simulink model "brasonduleur1"  (Simulink 7.9)
settings: Solver=ode1  StartTime=0.0  StopTime=1  RelTol=1e-3
libraries: powerlib x19, powerlib_extras x7, simulink_extras x1
settings Model: Creator=LiberT  LastModifiedBy=LiberT

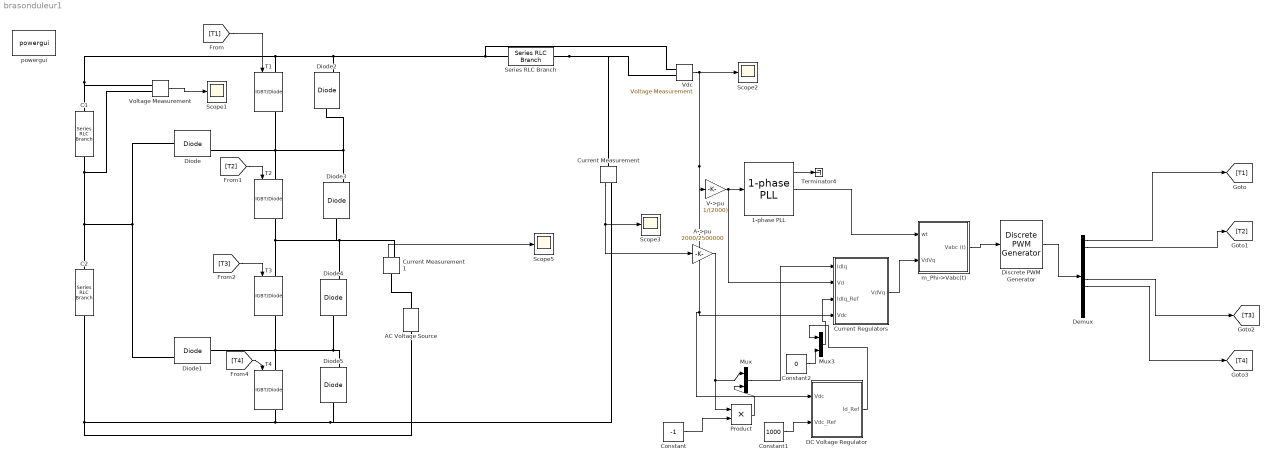
== system brasonduleur1 ==
  1-phase PLL : powerlib_extras/Control  Blocks/1-phase PLL  Par_Init=[0 60]  ParK=[ 180 3200 1 ]  AGC=off
  A->pu : Gain  Gain=2000/2500000  SaturateOnIntegerOverflow=on  OutDataTypeStr=Inherit: Same as input  ParamDataTypeStr=Inherit: Same as input
  AC Voltage Source : powerlib/Electrical Sources/AC Voltage Source  Amplitude=2e3  Phase=0  Frequency=60  SampleTime=0  Measurements=None
  C1 : powerlib/Elements/Series RLC Branch  LConnTagsString=__new0  RConnTagsString=__new0  BranchType=C  Resistance=1  Inductance=1e-3  SetiL0=off  InitialCurrent=0  Capacitance=150e-5  Setx0=off  InitialVoltage=0  Measurements=None
  C2 : powerlib/Elements/Series RLC Branch  LConnTagsString=__new0  RConnTagsString=__new0  BranchType=C  Resistance=1  Inductance=1e-3  SetiL0=off  InitialCurrent=0  Capacitance=150e-5  Setx0=off  InitialVoltage=0  Measurements=None
  Constant : Constant  Value=-1
  Constant1 : Constant  Value=1000
  Constant2 : Constant  Value=0
  Current Regulators : Subsystem  mask(Current Regulators){Kp=0.3, Ki=20, Kd=0, TcD=0.2e-3, Par_Limits=[12 -12], Init=0, Ts=5e-6}
      mask prompts: Kp "Proportional gain (Kp):"; Ki "Integral gain (Ki):"; Kd "Derivative gain (Kd):"; TcD "Time constant for derivative (s):"; Par_Limits "Output limits: [ Upper   Lower ]"; Init "Output initial value:"; Ts "Sample time:"
      mask help:
      | Sign convention:
      | Id positive(+) flowing into converter ==> Converter absorbing real power = P positive(+)
      | Iq negative(-) flowing into converter (inductive current) ==> Converter absorbing reactive power = Q positive(+)
  Current Measurement : powerlib/Measurements/Current Measurement  PhasorSimulation=off  OutputType=Complex  PSBequivalent=0
  Current Measurement1 : powerlib/Measurements/Current Measurement  PhasorSimulation=off  OutputType=Complex  PSBequivalent=0
  DC Voltage Regulator : Subsystem  mask(DC Voltage regulator){Kp=0.015, Ki=1.6, Ts=5e-6}
      mask prompts: Kp "Proportional gain (Kp):"; Ki "Integral gain(Ki)"; Ts "Sample time:"
  Demux : Demux  Outputs=12
  Diode{,1..5} (6 alike) : powerlib/Power Electronics/Diode  Ron=0.001  Lon=0  Vf=0.8  IC=0  UseSnubber=off  Rs=500  Cs=250e-9  Measurements=on
  Discrete PWM Generator : powerlib_extras/Discrete  Control Blocks/Discrete PWM Generator  GeneratorMode="Double 3-arm  bridges (12 pulses)"  Fc=333  Ts=5e-6  Internal=off  mIndex=0.4  Freq=333  Phase=0
  Mux : Mux  Inputs=2
  Mux3 : Mux  Inputs=2
  Product : Product  RndMeth=Zero
  Scope{1..3,5} (4 alike) : Scope
      Scope1 settings: YMin=1037.25  YMax=1041.5
      Scope2 settings: YMin=-1750  YMax=2500
      Scope3 settings: YMin=0.0965  YMax=0.1015  SaveName=ScopeData2
      Scope5 settings: YMin=-27500  YMax=2500  SaveName=ScopeData4
  Series RLC Branch : powerlib/Elements/Series RLC Branch  LConnTagsString=__new0  RConnTagsString=__new0  BranchType=RL  Resistance=1.25  Inductance=1  SetiL0=off  InitialCurrent=0  Capacitance=0  Setx0=off  InitialVoltage=0  Measurements=None
  T{1..4} (4 alike) : powerlib/Power Electronics/IGBT//Diode  Ron=0.2e-3  Rs=50  Cs=1e-6  Measurements=on
  Terminator4 : Terminator
  V->pu : Gain  Gain=1/(2000)  SaturateOnIntegerOverflow=on  OutDataTypeStr=Inherit: Same as input  ParamDataTypeStr=Inherit: Same as input
  Vdc : powerlib/Measurements/Voltage Measurement  PhasorSimulation=off  OutputType=Complex  PSBequivalent=0
  Voltage Measurement : powerlib/Measurements/Voltage Measurement  PhasorSimulation=off  OutputType=Complex  PSBequivalent=0
  m_Phi->Vabc(t) : Subsystem
  powergui : powerlib/powergui  Priority=1  SimulationMode=Discrete  SolverType=Tustin  SampleTime=50e-7  frequency=60  SPID=off  DisableSnubberDevices=off  DisableRonSwitches=off  DisableVfSwitches=off  SwTol=0  Interpol=off  DisplayEquations=off  FunctionMessages=off  frequencyindice=0  Pbase=100e6  ErrMax=1e-4  Iterations=50  UnitsV=kV  UnitsW=MW  echomessages=off  HookPort=off  EnableUseOfTLC=off  x0status=blocks  RestoreLinks=warning  ResistiveCurrentMeasurement=off  Ylog=off  Xlog=on  ShowGrid=off  save=off  variable=ZData  ZoomFFT=off  StartTime=0.0  cycles=1  DisplayStyle=1  FreqAxis=off  MaxFrequency=1000  frequencyindicesteady=1  display=off  methode=off
  wires:
  [T4] -> T4/1
  [T2] -> T2/1
  [T1] -> T1/1
  [T3] -> T3/1
  Voltage Measurement/1 -> Scope1/1
  Demux/2 -> [T2]
  Demux/8 -> [T4]
  Demux/7 -> [T3]
  Vdc/1 -> Scope2/1, V->pu/1, Current Regulators/4(Vdc), DC Voltage Regulator/1(Vdc)
  Current Measurement/1 -> Scope3/1, A->pu/1
  Demux/1 -> [T1]
  V->pu/1 -> 1-phase PLL/1, Current Regulators/2(Vd)
  1-phase PLL/1 -> Terminator4/1
  A->pu/1 -> Product/1, Mux/1
  Constant/1 -> Product/2
  Product/1 -> Mux/2
  Mux/1 -> Current Regulators/1(IdIq)
  Constant1/1 -> DC Voltage Regulator/2(Vdc_Ref)
  Constant2/1 -> Mux3/2
  DC Voltage Regulator/1(Id_Ref) -> Mux3/1
  Mux3/1 -> Current Regulators/3(IdIq_Ref)
  Current Regulators/1(VdVq) -> m_Phi->Vabc(t)/2(VdVq)
  1-phase PLL/2 -> m_Phi->Vabc(t)/1(wt)
  m_Phi->Vabc(t)/1(Vabc (t)) -> Discrete PWM Generator/1
  Current Measurement1/1 -> Scope5/1
  Discrete PWM Generator/1 -> Demux/1
  connections:
  Diode5/RConn1 -- T3/RConn1 -- T4/LConn1 -- Diode1/LConn1 -- Diode4/LConn1
  T1/RConn1 -- T2/LConn1 -- Diode/RConn1 -- Diode3/RConn1 -- Diode2/LConn1
  Series RLC Branch/LConn1 -- Vdc/LConn1 -- Diode2/RConn1 -- C1/LConn1 -- Voltage Measurement/LConn1 -- T1/LConn1
  C2/RConn1 -- T4/RConn1 -- Diode5/LConn1 -- Current Measurement/RConn1 -- AC Voltage Source/LConn1
  C1/RConn1 -- C2/LConn1 -- Diode1/RConn1 -- Diode/LConn1 -- Voltage Measurement/LConn2
  Series RLC Branch/RConn1 -- Current Measurement/LConn1 -- Vdc/LConn2
  T2/RConn1 -- T3/LConn1 -- Current Measurement1/RConn1 -- Diode4/RConn1 -- Diode3/LConn1
  AC Voltage Source/RConn1 -- Current Measurement1/LConn1

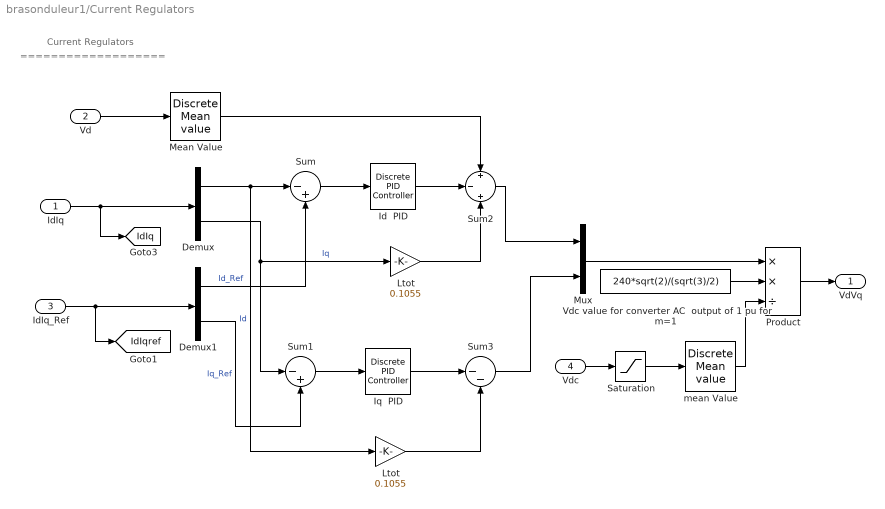
== system brasonduleur1/Current Regulators ==
  note: ===================
  note: Current Regulators
  IdIq : Inport  PortDimensions=2
  Vd : Inport  Port=2
  IdIq_Ref : Inport  Port=3  PortDimensions=2
  Vdc : Inport  Port=4
  " Ltot" : Gain  Gain=0.1055  SaturateOnIntegerOverflow=on  OutDataTypeStr=Inherit: Same as input  ParamDataTypeStr=Inherit: Same as input
  Demux : Demux  Outputs=2
  Demux1 : Demux  Outputs=2
  Id  PID : powerlib_extras/Discrete  Control Blocks/Discrete PID Controller  Kp=Kp  Ki=Ki  Kd=Kd  TcD=TcD  Par_Limits=Par_Limits  Init=Init  Ts=Ts
  Iq  PID : powerlib_extras/Discrete  Control Blocks/Discrete PID Controller  Kp=Kp  Ki=Ki  Kd=Kd  TcD=TcD  Par_Limits=Par_Limits  Init=Init  Ts=Ts
  "Ltot " : Gain  Gain=0.1055  SaturateOnIntegerOverflow=on  OutDataTypeStr=Inherit: Same as input  ParamDataTypeStr=Inherit: Same as input
  Mean Value : powerlib_extras/Discrete Measurements/Discrete  Mean value  Freq=60  Vinit=1.007  Ts=Ts
  Mux : Mux  Inputs=2
  Product : Product  Inputs=**/  SaturateOnIntegerOverflow=on  InputSameDT=on  OutDataTypeStr=Inherit: Same as first input
  Saturation : Saturate  UpperLimit=10000  LowerLimit=10
  Sum : Sum  Inputs=|-+  SaturateOnIntegerOverflow=on  InputSameDT=on  OutDataTypeStr=Inherit: Same as first input
  Sum1 : Sum  Inputs=|-+  SaturateOnIntegerOverflow=on  InputSameDT=on  OutDataTypeStr=Inherit: Same as first input
  Sum2 : Sum  Inputs=+|-|+  SaturateOnIntegerOverflow=on  InputSameDT=on  OutDataTypeStr=Inherit: Same as first input
  Sum3 : Sum  Inputs=|--  SaturateOnIntegerOverflow=on  InputSameDT=on  OutDataTypeStr=Inherit: Same as first input
  Vdc value for converter AC  output of 1 pu for m=1 : Constant  Value=240*sqrt(2)/(sqrt(3)/2)
  "mean Value " : powerlib_extras/Discrete Measurements/Discrete  Mean value  Freq=60  Vinit=500  Ts=Ts
  VdVq : Outport
  tag scope: IdIq=global, IdIqref=global
  wires:
  Sum3/1 -> Mux/2
  Vdc/1 -> Saturation/1
  "mean Value "/1 -> Product/3
  Vdc value for converter AC  output of 1 pu for m=1/1 -> Product/2
  Saturation/1 -> "mean Value "/1
  Mean Value/1 -> Sum2/1
  Product/1 -> VdVq/1
  IdIq_Ref/1 -> [IdIqref], Demux1/1
  Mux/1 -> Product/1
  Sum/1 -> Id  PID/1
  Demux1/2 -> Sum1/2  "Iq_Ref"
  Sum1/1 -> Iq  PID/1
  Demux/2 -> Sum1/1, "Ltot "/1  "Iq"
  Demux1/1 -> Sum/2  "Id_Ref"
  Demux/1 -> " Ltot"/1, Sum/1  "Id"
  IdIq/1 -> [IdIq], Demux/1
  Id  PID/1 -> Sum2/2
  Sum2/1 -> Mux/1
  Iq  PID/1 -> Sum3/1
  "Ltot "/1 -> Sum2/3
  " Ltot"/1 -> Sum3/2
  Vd/1 -> Mean Value/1

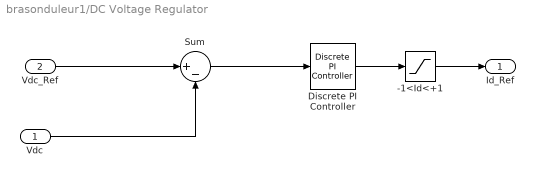
== system brasonduleur1/DC Voltage Regulator ==
  Vdc : Inport
  Vdc_Ref : Inport  Port=2
  -1<Id<+1 : Saturate  UpperLimit=1.2  LowerLimit=-1.2
  Discrete PI Controller : powerlib_extras/Discrete  Control Blocks/Discrete PI Controller  Kp=Kp  Ki=Ki  Par_Limits=[1.2 -1.2]  Init=0  Ts=Ts
  Sum : Sum  Inputs=|+-  SaturateOnIntegerOverflow=on  InputSameDT=on  OutDataTypeStr=Inherit: Same as first input
  Id_Ref : Outport  InitialOutput=0
  wires:
  Sum/1 -> Discrete PI Controller/1
  Vdc/1 -> Sum/2
  Discrete PI Controller/1 -> -1<Id<+1/1
  -1<Id<+1/1 -> Id_Ref/1
  Vdc_Ref/1 -> Sum/1

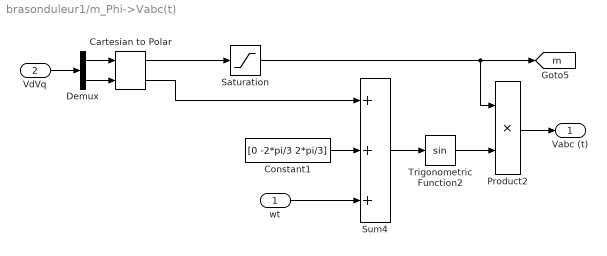
== system brasonduleur1/m_Phi->Vabc(t) ==
  wt : Inport
  VdVq : Inport  Port=2
  Cartesian to Polar : simulink_extras/Transformations/Cartesian to Polar
  Constant1 : Constant  Value=[0 -2*pi/3 2*pi/3]
  Demux : Demux  Outputs=2
  Product2 : Product  SaturateOnIntegerOverflow=on  InputSameDT=on  OutDataTypeStr=Inherit: Same as first input
  Saturation : Saturate  UpperLimit=1  LowerLimit=0
  Sum4 : Sum  Inputs=+++  SaturateOnIntegerOverflow=on  InputSameDT=on  OutDataTypeStr=Inherit: Same as first input
  Trigonometric Function2 : Trigonometry
  Vabc (t) : Outport
  tag scope: m=global
  wires:
  Saturation/1 -> [m], Product2/1
  Cartesian to Polar/1 -> Saturation/1
  Trigonometric Function2/1 -> Product2/2
  Sum4/1 -> Trigonometric Function2/1
  Cartesian to Polar/2 -> Sum4/1
  Demux/2 -> Cartesian to Polar/2
  Demux/1 -> Cartesian to Polar/1
  VdVq/1 -> Demux/1
  wt/1 -> Sum4/3
  Product2/1 -> Vabc (t)/1
  Constant1/1 -> Sum4/2
